simulink model "FDI_and_sensors"  (R2021b)
settings: Solver=VariableStepAuto  StartTime=0.0  StopTime=10.0  RelTol=1e-3
values from neighbouring files (symbols this model uses):
  aoa_sensor_measurement_limit_rad = deg2rad(30)    [init_sensor_model.m]
  aoa_sensor_noise_power = 0.00030462    [init_sensor_model.m]
  bias_fault_active = TRUE    (= 1)    [fault_configurations.m]
  bias_fault_time = 150    [fault_configurations.m]
  bias_rad = deg2rad(3)    [fault_configurations.m]
  drift_fault_active = FALSE    (= 0)    [fault_configurations.m]
  drift_limit_rad = deg2rad(20)    [fault_configurations.m]
  drift_ratio_rad_s = deg2rad(0.2)    [fault_configurations.m]
  dt = 1/50    (= 0.02)    [aerosonde_initialize.m]
  stuck_fault_active = FALSE    (= 0)    [fault_configurations.m]
undefined symbols (not defined in the file or in its folder): m, s
libraries: simulink_extras x14, simulink x2, aerolibconvert2 x1
settings Model: Creator=altin  LastModifiedBy=altin

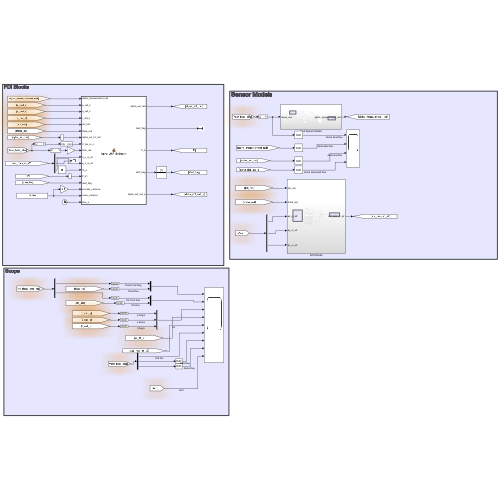
[thumbnail: Simulink's stored preview of the top-level diagram]
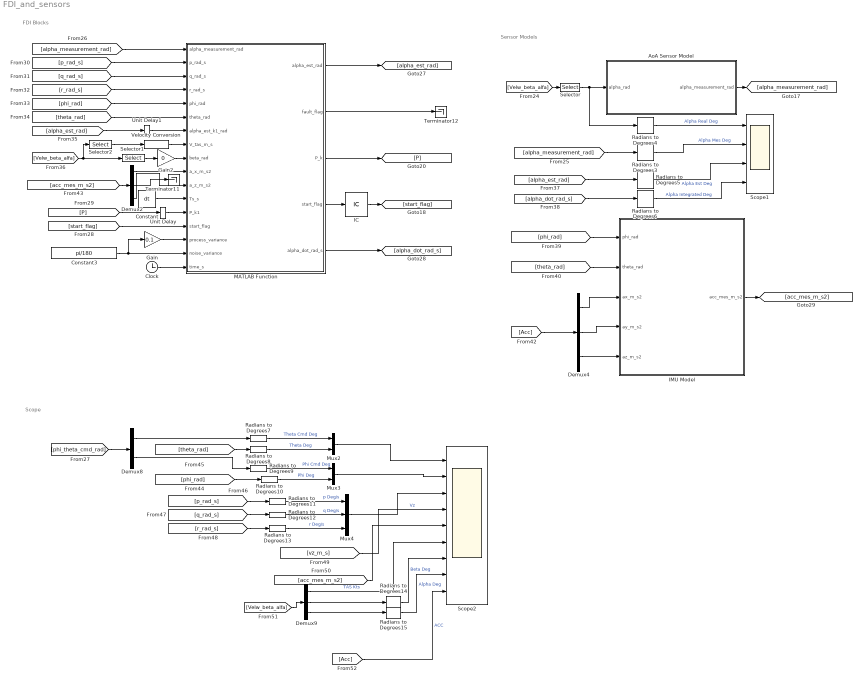
== system FDI_and_sensors ==
  note: Scope
  note: FDI Blocks
  note: Sensor Models
  AoA Sensor Model : Subsystem
  Clock : Clock
  Constant : Constant  Value=dt
  Constant3 : Constant  Value=pi/180
  Demux2 : Demux  Outputs=3
  Demux4 : Demux  Outputs=3
  Demux8 : Demux  Outputs=2
  Demux9 : Demux  Outputs=3
  Gain : Gain  Gain=0.1
  Gain2 : Gain  Gain=0
  IC : InitialCondition
  IMU Model : Subsystem
  MATLAB Function : MATLAB Function  TreatAsAtomicUnit=on
  Mux2 : Mux  Inputs=2
  Mux3 : Mux  Inputs=2
  Mux4 : Mux  Inputs=3
  Radians to Degrees{3..15} (13 alike) : simulink_extras/Transformations/Radians to Degrees
  Scope1 : Scope  NumInputPorts=4
  Scope2 : Scope  NumInputPorts=9
  Selector : Selector  InputPortWidth=3  IndexOptions=Index vector (dialog)  Indices=[3]  OutputSizes=1
  Selector1 : Selector  InputPortWidth=3  IndexOptions=Index vector (dialog)  Indices=[2]  OutputSizes=1
  Selector2 : Selector  InputPortWidth=3  IndexOptions=Index vector (dialog)  Indices=[1]  OutputSizes=1
  Terminator11 : Terminator
  Terminator12 : Terminator
  Unit Delay : UnitDelay  SampleTime=-1  HasFrameUpgradeWarning=on
  Unit Delay1 : UnitDelay  SampleTime=-1  HasFrameUpgradeWarning=on
  Velocity Conversion : aerolibconvert2/Velocity Conversion  IU=kts  OU=m/s
  wires:
  Radians to Degrees14/1 -> Scope2/7  "Beta Deg"
  [Velw_beta_alfa] -> Demux9/1
  Clock/1 -> MATLAB Function/17(time_s)
  Mux3/1 -> Scope2/2
  Demux9/3 -> Radians to Degrees15/1
  Gain2/1 -> MATLAB Function/9(beta_rad)
  Radians to Degrees15/1 -> Scope2/8  "Alpha Deg"
  Radians to Degrees10/1 -> Mux3/2  "Phi Deg"
  Demux2/3 -> MATLAB Function/11(a_z_m_s2)
  [r_rad_s] -> Radians to Degrees13/1
  [q_rad_s] -> Radians to Degrees12/1
  Gain/1 -> MATLAB Function/15(process_variance)
  [phi_theta_cmd_rad] -> Demux8/1
  [theta_rad] -> Radians to Degrees8/1
  Constant/1 -> MATLAB Function/12(Ts_s)
  Demux2/1 -> MATLAB Function/10(a_x_m_s2)
  MATLAB Function/2(fault_flag) -> Terminator12/1
  Unit Delay/1 -> MATLAB Function/13(P_k1)
  [q_rad_s] -> MATLAB Function/3(q_rad_s)
  [p_rad_s] -> Radians to Degrees11/1
  MATLAB Function/1(alpha_est_rad) -> [alpha_est_rad]
  Demux2/2 -> Terminator11/1
  [theta_rad] -> MATLAB Function/6(theta_rad)
  [alpha_measurement_rad] -> MATLAB Function/1(alpha_measurement_rad)
  [acc_mes_m_s2] -> Demux2/1
  [Velw_beta_alfa] -> Selector1/1, Selector2/1
  MATLAB Function/4(start_flag) -> IC/1
  [acc_mes_m_s2] -> Scope2/5
  Radians to Degrees13/1 -> Mux4/3  "r Deg/s"
  Mux4/1 -> Scope2/3
  Demux9/1 -> Scope2/6  "TAS Kts"
  Velocity Conversion/1 -> MATLAB Function/8(V_tas_m_s)
  [p_rad_s] -> MATLAB Function/2(p_rad_s)
  Radians to Degrees9/1 -> Mux3/1  "Phi Cmd Deg"
  Selector2/1 -> Velocity Conversion/1
  Unit Delay1/1 -> MATLAB Function/7(alpha_est_k1_rad)
  IC/1 -> [start_flag]
  MATLAB Function/3(P_k) -> [P]
  Demux8/2 -> Radians to Degrees9/1
  Radians to Degrees8/1 -> Mux2/2  "Theta Deg"
  [P] -> Unit Delay/1
  [phi_rad] -> MATLAB Function/5(phi_rad)
  [r_rad_s] -> MATLAB Function/4(r_rad_s)
  [start_flag] -> MATLAB Function/14("start_flag ")
  Radians to Degrees7/1 -> Mux2/1  "Theta Cmd Deg"
  Constant3/1 -> Gain/1, MATLAB Function/16(noise_variance)
  Demux9/2 -> Radians to Degrees14/1
  Selector1/1 -> Gain2/1
  Demux8/1 -> Radians to Degrees7/1
  [Acc] -> Scope2/9  "ACC"
  [vz_m_s] -> Scope2/4  "Vz"
  [alpha_est_rad] -> Unit Delay1/1
  MATLAB Function/5(alpha_dot_rad_s) -> [alpha_dot_rad_s]
  Radians to Degrees12/1 -> Mux4/2  "q Deg/s"
  Radians to Degrees11/1 -> Mux4/1  "p Deg/s"
  Mux2/1 -> Scope2/1
  [phi_rad] -> Radians to Degrees10/1
  [theta_rad] -> IMU Model/2(theta_rad)
  [phi_rad] -> IMU Model/1(phi_rad)
  Demux4/1 -> IMU Model/3(ax_m_s2)
  Radians to Degrees6/1 -> Scope1/4  "Alpha Integrated Deg"
  [Acc] -> Demux4/1
  Demux4/2 -> IMU Model/4(ay_m_s2)
  Demux4/3 -> IMU Model/5(az_m_s2)
  [alpha_dot_rad_s] -> Radians to Degrees6/1
  [alpha_est_rad] -> Radians to Degrees5/1
  Radians to Degrees5/1 -> Scope1/3  "Alpha Est Deg"
  [alpha_measurement_rad] -> Radians to Degrees3/1
  Radians to Degrees3/1 -> Scope1/2  "Alpha Mes Deg"
  AoA Sensor Model/1(alpha_measurement_rad) -> [alpha_measurement_rad]
  Radians to Degrees4/1 -> Scope1/1  "Alpha Real Deg"
  Selector/1 -> Radians to Degrees4/1, AoA Sensor Model/1(alpha_rad)
  IMU Model/1(acc_mes_m_s2) -> [acc_mes_m_s2]
  [Velw_beta_alfa] -> Selector/1

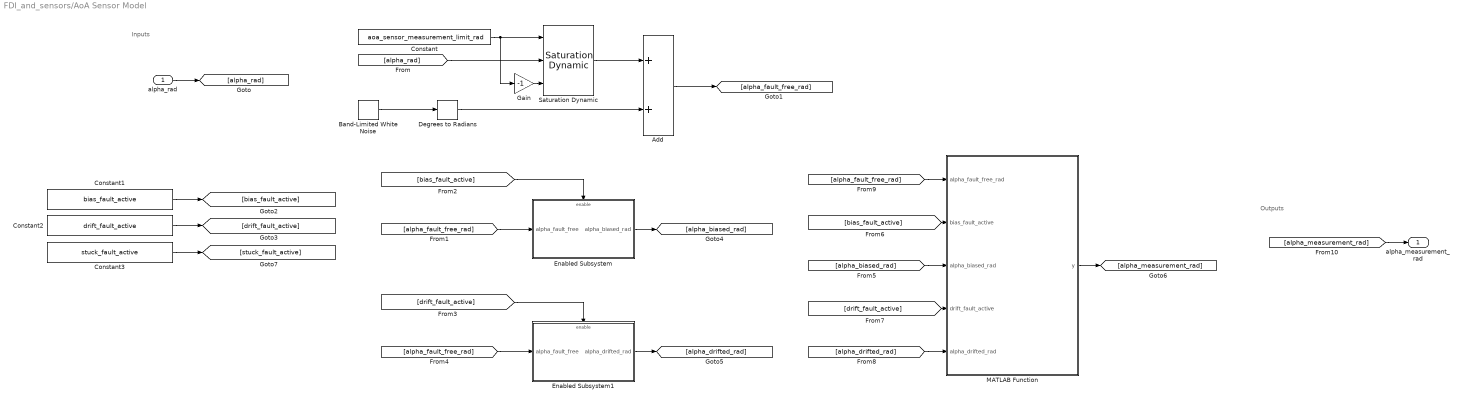
== system FDI_and_sensors/AoA Sensor Model ==
  note: Outputs
  note: Inputs
  alpha_rad : Inport
  Add : Sum
  Band-Limited White Noise : simulink/Sources/Band-Limited White Noise  Cov=[aoa_sensor_noise_power]  Ts=dt  seed=[23341]
  Constant : Constant  Value=aoa_sensor_measurement_limit_rad
  Constant1 : Constant  Value=bias_fault_active
  Constant2 : Constant  Value=drift_fault_active
  Constant3 : Constant  Value=stuck_fault_active
  Degrees to Radians : simulink_extras/Transformations/Degrees to Radians
  Enabled Subsystem : Subsystem  TreatAsAtomicUnit=on
  Enabled Subsystem1 : Subsystem  TreatAsAtomicUnit=on
  Gain : Gain  Gain=-1
  MATLAB Function : MATLAB Function  TreatAsAtomicUnit=on
  Saturation Dynamic : simulink/Discontinuities/Saturation Dynamic  OutMin=[]  OutMax=[]  OutDataTypeStr=Inherit: Same as second input  OutDataType=fixdt(1, 16)  OutScaling=2^-10  DoSatur=off
  alpha_measurement_rad : Outport
  wires:
  alpha_rad/1 -> [alpha_rad]
  [alpha_rad] -> Saturation Dynamic/2
  Gain/1 -> Saturation Dynamic/3
  Constant/1 -> Saturation Dynamic/1, Gain/1
  Saturation Dynamic/1 -> Add/1
  Band-Limited White Noise/1 -> Degrees to Radians/1
  Add/1 -> [alpha_fault_free_rad]
  Constant1/1 -> [bias_fault_active]
  Constant2/1 -> [drift_fault_active]
  [bias_fault_active] -> Enabled Subsystem/Enable
  [alpha_fault_free_rad] -> Enabled Subsystem/1(alpha_fault_free)
  [drift_fault_active] -> Enabled Subsystem1/Enable
  [alpha_fault_free_rad] -> Enabled Subsystem1/1(alpha_fault_free)
  Enabled Subsystem/1(alpha_biased_rad) -> [alpha_biased_rad]
  Enabled Subsystem1/1(alpha_drifted_rad) -> [alpha_drifted_rad]
  [alpha_biased_rad] -> MATLAB Function/3(alpha_biased_rad)
  [bias_fault_active] -> MATLAB Function/2(bias_fault_active)
  [drift_fault_active] -> MATLAB Function/4(drift_fault_active)
  [alpha_drifted_rad] -> MATLAB Function/5(alpha_drifted_rad)
  [alpha_fault_free_rad] -> MATLAB Function/1(alpha_fault_free_rad)
  MATLAB Function/1(y) -> [alpha_measurement_rad]
  [alpha_measurement_rad] -> alpha_measurement_rad/1
  Degrees to Radians/1 -> Add/2
  Constant3/1 -> [stuck_fault_active]

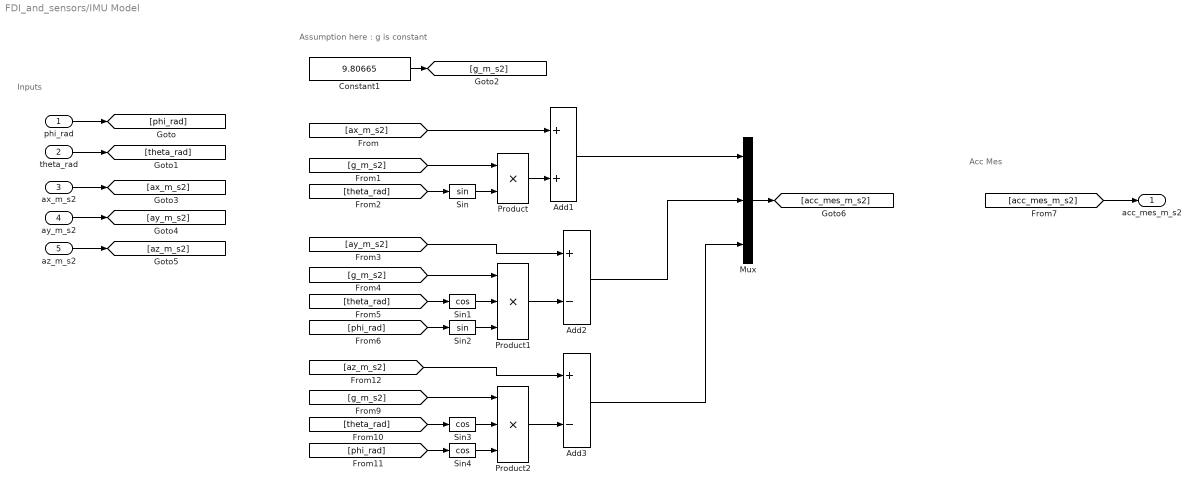
== system FDI_and_sensors/IMU Model ==
  note: Assumption here : g is constant
  note: Acc Mes
  note: Inputs
  phi_rad : Inport
  theta_rad : Inport  Port=2
  ax_m_s2 : Inport  Port=3
  ay_m_s2 : Inport  Port=4
  az_m_s2 : Inport  Port=5
  Add1 : Sum
  Add2 : Sum  Inputs=+-
  Add3 : Sum  Inputs=+-
  Constant1 : Constant  Value=9.80665
  Mux : Mux  Inputs=3
  Product : Product
  Product1 : Product  Inputs=3
  Product2 : Product  Inputs=3
  Sin : Trigonometry
  Sin1 : Trigonometry  Operator=cos
  Sin2 : Trigonometry
  Sin3 : Trigonometry  Operator=cos
  Sin4 : Trigonometry  Operator=cos
  acc_mes_m_s2 : Outport
  wires:
  phi_rad/1 -> [phi_rad]
  theta_rad/1 -> [theta_rad]
  az_m_s2/1 -> [az_m_s2]
  ay_m_s2/1 -> [ay_m_s2]
  ax_m_s2/1 -> [ax_m_s2]
  [acc_mes_m_s2] -> acc_mes_m_s2/1
  Constant1/1 -> [g_m_s2]
  [g_m_s2] -> Product/1
  Sin/1 -> Product/2
  [theta_rad] -> Sin/1
  Product/1 -> Add1/2
  [ax_m_s2] -> Add1/1
  Add1/1 -> Mux/1
  Mux/1 -> [acc_mes_m_s2]
  [g_m_s2] -> Product1/1
  [theta_rad] -> Sin1/1
  Sin1/1 -> Product1/2
  [phi_rad] -> Sin2/1
  Sin2/1 -> Product1/3
  Product1/1 -> Add2/2
  [ay_m_s2] -> Add2/1
  [az_m_s2] -> Add3/1
  Product2/1 -> Add3/2
  Sin4/1 -> Product2/3
  [phi_rad] -> Sin4/1
  Sin3/1 -> Product2/2
  [theta_rad] -> Sin3/1
  [g_m_s2] -> Product2/1
  Add2/1 -> Mux/2
  Add3/1 -> Mux/3

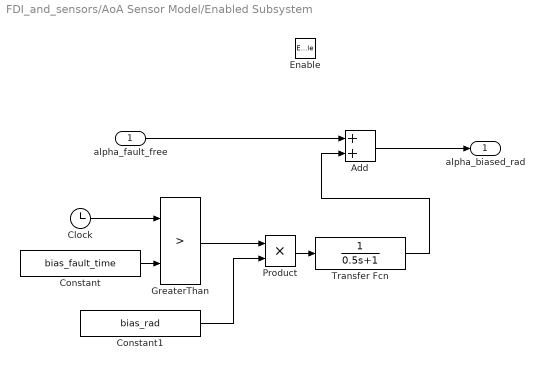
== system FDI_and_sensors/AoA Sensor Model/Enabled Subsystem ==
  alpha_fault_free : Inport
  Enable : EnablePort
  Add : Sum
  Clock : Clock
  Constant : Constant  Value=bias_fault_time
  Constant1 : Constant  Value=bias_rad
  GreaterThan : RelationalOperator  Operator=>  OutDataTypeStr=boolean  RndMeth=Simplest
  Product : Product
  Transfer Fcn : TransferFcn  Denominator=[0.5 1]
  alpha_biased_rad : Outport
  wires:
  Clock/1 -> GreaterThan/1
  Constant/1 -> GreaterThan/2
  GreaterThan/1 -> Product/1
  Constant1/1 -> Product/2
  Product/1 -> Transfer Fcn/1
  alpha_fault_free/1 -> Add/1
  Transfer Fcn/1 -> Add/2
  Add/1 -> alpha_biased_rad/1

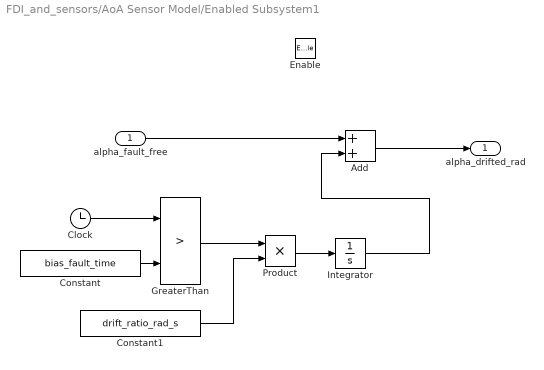
== system FDI_and_sensors/AoA Sensor Model/Enabled Subsystem1 ==
  alpha_fault_free : Inport
  Enable : EnablePort
  Add : Sum
  Clock : Clock
  Constant : Constant  Value=bias_fault_time
  Constant1 : Constant  Value=drift_ratio_rad_s
  GreaterThan : RelationalOperator  Operator=>  OutDataTypeStr=boolean  RndMeth=Simplest
  Integrator : Integrator  LimitOutput=on  UpperSaturationLimit=drift_limit_rad  LowerSaturationLimit=-drift_limit_rad
  Product : Product
  alpha_drifted_rad : Outport
  wires:
  Add/1 -> alpha_drifted_rad/1
  Integrator/1 -> Add/2
  alpha_fault_free/1 -> Add/1
  Product/1 -> Integrator/1
  Constant1/1 -> Product/2
  GreaterThan/1 -> Product/1
  Constant/1 -> GreaterThan/2
  Clock/1 -> GreaterThan/1

== matlab function FDI_and_sensors/AoA Sensor Model/MATLAB Function ==
  data: alpha_fault_free_rad input; y output; bias_fault_active input; alpha_biased_rad input; drift_fault_active input; alpha_drifted_rad input
function y = fcn(alpha_fault_free_rad, ...
                 bias_fault_active, ...
                 alpha_biased_rad,...
                 drift_fault_active,...
                 alpha_drifted_rad)
TRUE = 1;
FALSE = 0;

if((TRUE  == bias_fault_active ) &&...
   (FALSE == drift_fault_active)  )
    y = alpha_biased_rad;

elseif((FALSE == bias_fault_active ) &&...
       (TRUE == drift_fault_active )  )
    y = alpha_drifted_rad;
else
    y = alpha_fault_free_rad;
end

== matlab function FDI_and_sensors/MATLAB Function ==
  data: alpha_measurement_rad input; p_rad_s input; q_rad_s input; r_rad_s input; phi_rad input; theta_rad input; alpha_est_k1_rad input; V_tas_m_s input; beta_rad input; a_x_m_s2 input; a_z_m_s2 input; Ts_s input; P_k1 input; alpha_est_rad output; fault_flag output; P_k output; start_flag input; start_flag output; process_variance input; noise_variance input; alpha_dot_rad_s output; time_s input
function [alpha_est_rad, fault_flag,P_k,start_flag,alpha_dot_rad_s] = Alpha_UKF_Estimator(alpha_measurement_rad,...
                                                           p_rad_s,q_rad_s, r_rad_s,...
                                                           phi_rad, theta_rad, ...
                                                           alpha_est_k1_rad, V_tas_m_s, ...
                                                           beta_rad, ...
                                                           a_x_m_s2,a_z_m_s2, ...
                                                           Ts_s, P_k1, ...
                                                           start_flag, ...
                                                           process_variance, ...
                                                           noise_variance, ...
                                                           time_s)
    
    TRUE  = 1;
    FALSE = 0;
    standby_time_s = 50;
    
    if(time_s<standby_time_s)
        start_flag = FALSE;
        P_k1 = 1;
    end
 
    Q = process_variance^2;
    R = noise_variance^2;  

    %% Prediction step
    g_m_s2  = 9.80665;
    c_phi   = cos(phi_rad      );
    c_theta = cos(theta_rad    );
    c_alpha = cos(alpha_est_k1_rad);

    s_theta = sin(theta_rad);
    s_alpha = sin(alpha_est_k1_rad);
    c_beta  = cos(beta_rad);

    t_beta  = tan(beta_rad);

    alpha_dot_rad_s = q_rad_s + ...
                     (g_m_s2*c_phi*c_theta*c_alpha + g_m_s2*s_theta*s_alpha - ...
                      a_x_m_s2*s_alpha + a_z_m_s2*c_alpha) / (V_tas_m_s * c_beta) - ...
                      (p_rad_s * c_alpha + r_rad_s * s_alpha) * t_beta;

    alpha_pred_rad = alpha_est_k1_rad + alpha_dot_rad_s * Ts_s;

    % Sytem Jacobian
    F =  (g_m_s2*c_phi*c_theta*-1*s_alpha + g_m_s2*s_theta*c_alpha - ...
          -1* a_x_m_s2*c_alpha - a_z_m_s2*s_alpha) / (V_tas_m_s * c_beta) - ...
          (r_rad_s * c_alpha - p_rad_s * s_alpha) * t_beta;

    % Error Covariance Matrix
    P_k = F * P_k1 * F + Q;

    % Kalman Gain
    K = P_k*(P_k + R)^(-1);

    %% Update Step
    alpha_est_rad = alpha_pred_rad + K*(alpha_measurement_rad - alpha_pred_rad);
    P_k = (1 - K)* P_k;

    %% Residual
    fault_flag = FALSE;








end
